simulink model "Ven_mac_Melay"  (R2020b)
settings: Solver=VariableStepAuto  StartTime=0.0  StopTime=1  RelTol=1e-3
settings Model: Creator=Eshan  LastModifiedBy=Eshan

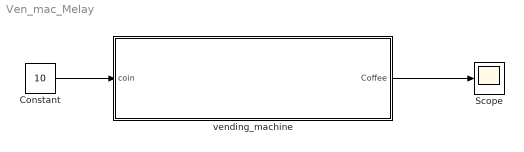
== system Ven_mac_Melay ==
  Constant : Constant  Value=10
  Scope : Scope
  vending_machine : Stateflow chart  TreatAsAtomicUnit=on
  wires:
  vending_machine/1(Coffee) -> Scope/1
  Constant/1 -> vending_machine/1(coin)

== stateflow chart Ven_mac_Melay/vending_machine ==
  state got_0
    entry:
    Coffee=0;
  state got_20rs
    entry:
    Coffee=1;
  state got_10rs
    entry:
    Coffee=0;
  (default) -> got_0
  got_0 -> got_20rs [order 1] : [coin==10]{Coffee==0}
  got_20rs -> got_0 [order 1] : [coin==20]{Coffee==1}
  got_0 -> got_10rs [order 2] : [coin==20]{Coffee==0}
  got_10rs -> got_0 [order 1] : [coin==10]{Coffee==1}
  got_20rs -> got_10rs [order 2] : [coin==10]{Coffee==0}
  got_10rs -> got_20rs [order 2] : [coin==20]{Coffee==1}
  data: coin input size=1; Coffee output
